simulink model "firstorder"  (R2021b)
settings: Solver=ode23t  StartTime=0.0  StopTime=1  MaxStep=1e-6  RelTol=1e-3
settings Model: Creator=alexey  LastModifiedBy=alexey
settings SolverCC: ZeroCrossControl=DisableAll

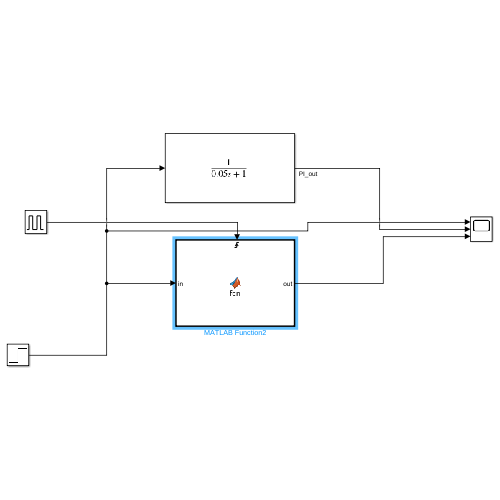
[thumbnail: Simulink's stored preview of the top-level diagram]
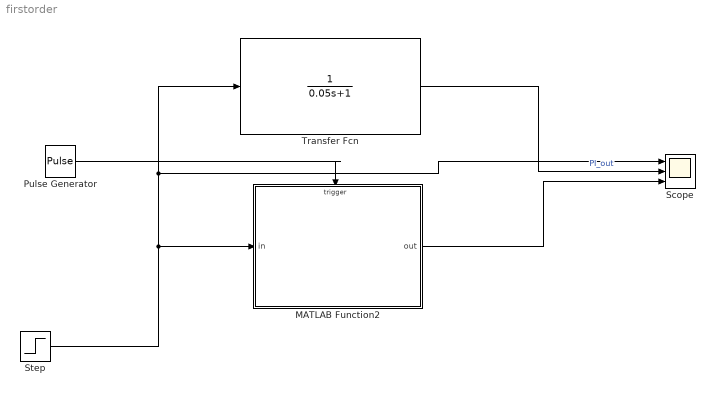
== system firstorder ==
  MATLAB Function2 : MATLAB Function  TreatAsAtomicUnit=on
  Pulse Generator : DiscretePulseGenerator  PulseType=Time based  Period=10e-6
  Scope : Scope  NumInputPorts=3
  Step : Step  Time=0.1  SampleTime=0
  Transfer Fcn : TransferFcn  Denominator=[0.05 1]
  wires:
  Pulse Generator/1 -> MATLAB Function2/Trigger
  Transfer Fcn/1 -> Scope/2  "PI_out"
  MATLAB Function2/1(out) -> Scope/3
  Step/1 -> MATLAB Function2/1(in), Scope/1, Transfer Fcn/1

== matlab function firstorder/MATLAB Function2 ==
  data: in input; out output
  events: trigger input RISING_EDGE_EVENT
function out = fcn(in)
dt = 10e-6;
alfa = 0.05;
persistent prev
if isempty(prev)
    prev = 0;
end

out = prev * (1 - dt*(1/alfa)) + ((1/alfa)*dt)* in;
prev = out;
end
